simulink model "ModDem_OFDM_multicamino"  (R2018a)
settings: Solver=FixedStepAuto  StartTime=0.0  StopTime=M*CantBit  FixedStep=Tsampling  RelTol=1e-3
values from neighbouring files (symbols this model uses):
  EsOFDM = 2    [Script_configParametros_multicamino.m]
  F1 = FsepOFDM*2    [Script_configParametros_multicamino.m]
  F2 = FsepOFDM*3    [Script_configParametros_multicamino.m]
  F3 = FsepOFDM*4    [Script_configParametros_multicamino.m]
  F4 = FsepOFDM*5    [Script_configParametros_multicamino.m]
  RbOFDM = RsOFDM*sum(TransfBitPerSimb)    [Script_configParametros_multicamino.m]
  Ts1 = Tb1    (= 0.04)    [Script_configParametros_multicamino.m]
  Ts2 = Tb2    (= 0.04)    [Script_configParametros_multicamino.m]
  Ts3 = Tb3    (= 0.04)    [Script_configParametros_multicamino.m]
  Ts4 = Tb4    (= 0.04)    [Script_configParametros_multicamino.m]
  Tsampling = M/N    [Script_configParametros_multicamino.m]
libraries: commdigbbndpm3 x8, dspsigops x8, simulink x1, commrandsrc3 x1
settings Model: Creator=lukit  LastModifiedBy=geroo
settings DebuggingCC: LibraryContextMissingDiagnostic=warning
settings SFSimCC: SimUseLocalCustomCode=on
settings RTWCC: RTWUseLocalCustomCode=on

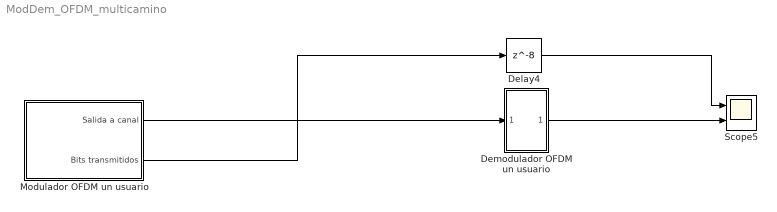
== system ModDem_OFDM_multicamino ==
  Delay4 : Delay  DelayLength=8  InitialCondition=0  InputProcessing=Columns as channels (frame based)
  Demodulador OFDM un usuario : Subsystem
  Modulador OFDM un usuario : Subsystem
  Scope5 : Scope  NumInputPorts=2
  wires:
  Modulador OFDM un usuario/2(Bits transmitidos) -> Delay4/1
  Delay4/1 -> Scope5/1
  Modulador OFDM un usuario/1(Salida a canal) -> Demodulador OFDM un usuario/1(In1)
  Demodulador OFDM un usuario/1(Out1) -> Scope5/2

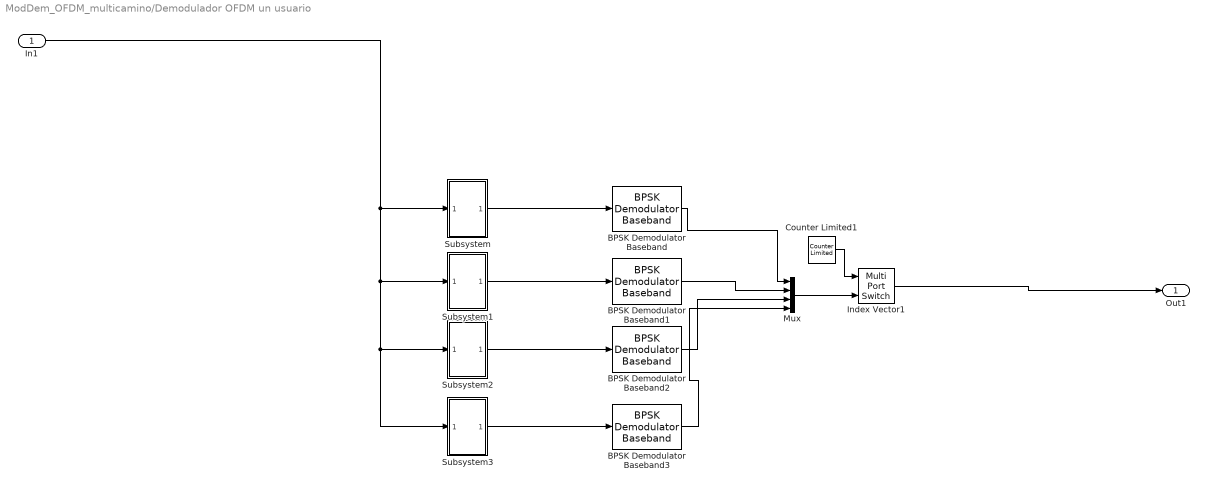
== system ModDem_OFDM_multicamino/Demodulador OFDM un usuario ==
  In1 : Inport
  BPSK Demodulator Baseband{,1..3} (4 alike) : commdigbbndpm3/BPSK Demodulator Baseband  DecType=Hard decision  VarSource=Dialog  Variance=1  Ph=0  outDtype=Inherit via internal rule  derotateFactorWordLen=16  derotateFactorDataTypeStr=Inherit: Same word length as input  derotateFactorLastDataTypeStr=Inherit: Same word length as input
  Counter Limited1 : simulink/Sources/Counter Limited  uplimit=3  tsamp=1/RbOFDM
  Index Vector1 : MultiPortSwitch  DataPortOrder=Zero-based contiguous  Inputs=1  zeroidx=on
  Mux : Mux
  Subsystem : Subsystem
  Subsystem1 : Subsystem
  Subsystem2 : Subsystem
  Subsystem3 : Subsystem
  Out1 : Outport
  wires:
  Subsystem1/1(Out1) -> BPSK Demodulator Baseband1/1
  Subsystem/1(Out1) -> BPSK Demodulator Baseband/1
  Index Vector1/1 -> Out1/1
  BPSK Demodulator Baseband3/1 -> Mux/4
  Subsystem2/1(Out1) -> BPSK Demodulator Baseband2/1
  In1/1 -> Subsystem3/1(In1), Subsystem2/1(In1), Subsystem1/1(In1), Subsystem/1(In1)
  BPSK Demodulator Baseband2/1 -> Mux/3
  BPSK Demodulator Baseband1/1 -> Mux/2
  BPSK Demodulator Baseband/1 -> Mux/1
  Mux/1 -> Index Vector1/2
  Subsystem3/1(Out1) -> BPSK Demodulator Baseband3/1
  Counter Limited1/1 -> Index Vector1/1

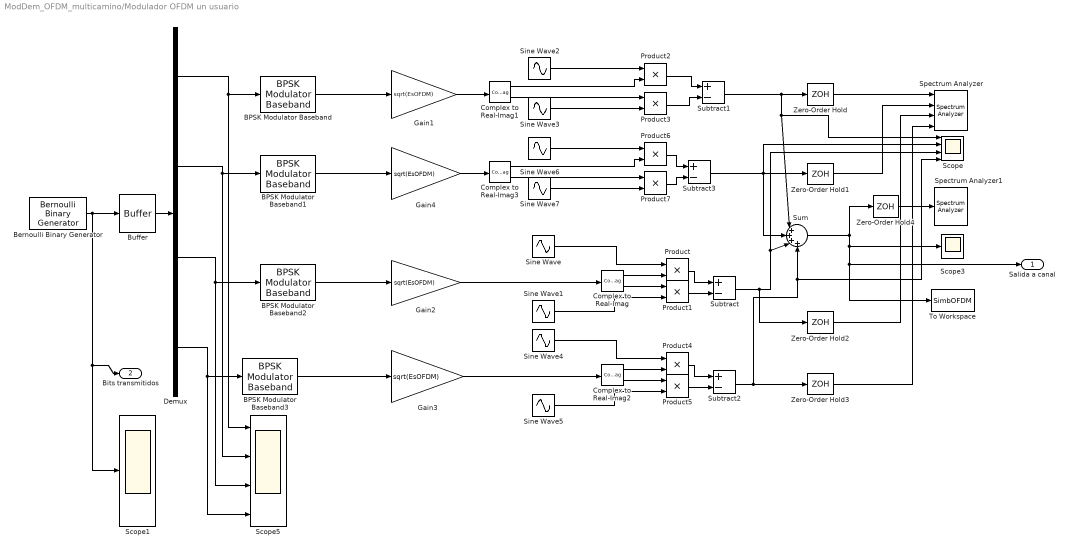
== system ModDem_OFDM_multicamino/Modulador OFDM un usuario ==
  BPSK Modulator Baseband{,1..3} (4 alike) : commdigbbndpm3/BPSK Modulator Baseband  Ph=0  outDtype=double  outWordLen=16  outUDDataType=sfix(16)  outFracLenMode=Best precision  outFracLen=15  outDataTypeStr=double  outLastDataTypeStr=double
  Bernoulli Binary Generator : commrandsrc3/Bernoulli Binary Generator  ProbabilityOfZero=0.5  SeedSource=Auto  Seed=0  SampleTime=1/RbOFDM  SamplesPerFrame=1  OutputDataType=double  SimulateUsing=Interpreted execution
  Buffer : Buffer  N=4  OutputFrames=off
  Complex to Real-Imag{,1..3} (4 alike) : ComplexToRealImag
  Demux : Demux
  Gain{1..4} (4 alike) : Gain  Gain=sqrt(EsOFDM)
  Product{,1..7} (8 alike) : Product
  Scope : Scope  NumInputPorts=4
  Scope1 : Scope
  Scope3 : Scope
  Scope5 : Scope  NumInputPorts=4
  Sine Wave : Sin  Amplitude=sqrt(2/Ts3)  Frequency=2*pi*F3  Phase=pi/2  SampleTime=Tsampling
  Sine Wave1 : Sin  Amplitude=sqrt(2/Ts3)  Frequency=2*pi*F3  SampleTime=Tsampling
  Sine Wave2 : Sin  Amplitude=sqrt(2/Ts1)  Frequency=2*pi*F1  Phase=pi/2  SampleTime=Tsampling
  Sine Wave3 : Sin  Amplitude=sqrt(2/Ts1)  Frequency=2*pi*F1  SampleTime=Tsampling
  Sine Wave4 : Sin  Amplitude=sqrt(2/Ts4)  Frequency=2*pi*F4  Phase=pi/2  SampleTime=Tsampling
  Sine Wave5 : Sin  Amplitude=sqrt(2/Ts4)  Frequency=2*pi*F4  SampleTime=Tsampling
  Sine Wave6 : Sin  Amplitude=sqrt(2/Ts2)  Frequency=2*pi*F2  Phase=pi/2  SampleTime=Tsampling
  Sine Wave7 : Sin  Amplitude=sqrt(2/Ts2)  Frequency=2*pi*F2  SampleTime=Tsampling
  Spectrum Analyzer : SpectrumAnalyzer  NumInputPorts=4
  Spectrum Analyzer1 : SpectrumAnalyzer
  Subtract{,1..3} (4 alike) : Sum  Inputs=+-
  Sum : Sum  Inputs=|++++
  To Workspace : ToWorkspace  VariableName=SimbOFDM  SampleTime=Tsampling
      settings: Save2DSignal=2-D array (concatenate along first dimension)
  Zero-Order Hold{,1..4} (5 alike) : ZeroOrderHold  SampleTime=-1
  Salida a canal : Outport
  Bits transmitidos : Outport  Port=2
  wires:
  BPSK Modulator Baseband/1 -> Gain1/1
  Zero-Order Hold1/1 -> Spectrum Analyzer/2
  Complex to Real-Imag3/2 -> Product7/1
  Gain4/1 -> Complex to Real-Imag3/1
  Sine Wave5/1 -> Product5/2
  Gain1/1 -> Complex to Real-Imag1/1
  Bernoulli Binary Generator/1 -> Bits transmitidos/1, Scope1/1, Buffer/1
  Product/1 -> Subtract/1
  Complex to Real-Imag2/2 -> Product5/1
  Subtract3/1 -> Zero-Order Hold1/1, Sum/2, Scope/2
  Product2/1 -> Subtract1/1
  Subtract2/1 -> Zero-Order Hold3/1, Scope/4, Sum/4
  Zero-Order Hold2/1 -> Spectrum Analyzer/3
  Complex to Real-Imag1/2 -> Product3/1
  Sine Wave3/1 -> Product3/2
  Zero-Order Hold3/1 -> Spectrum Analyzer/4
  Gain2/1 -> Complex to Real-Imag/1
  Sine Wave2/1 -> Product2/1
  Demux/3 -> BPSK Modulator Baseband2/1, Scope5/3
  Subtract1/1 -> Sum/1, Scope/1, Zero-Order Hold/1
  Subtract/1 -> Zero-Order Hold2/1, Scope/3, Sum/3
  Product4/1 -> Subtract2/1
  Product3/1 -> Subtract1/2
  Buffer/1 -> Demux/1
  Sum/1 -> Salida a canal/1, To Workspace/1, Scope3/1, Zero-Order Hold4/1
  Product1/1 -> Subtract/2
  Sine Wave4/1 -> Product4/1
  Demux/1 -> BPSK Modulator Baseband/1, Scope5/1
  Complex to Real-Imag2/1 -> Product4/2
  Complex to Real-Imag/1 -> Product/2
  Sine Wave1/1 -> Product1/2
  Product7/1 -> Subtract3/2
  Zero-Order Hold4/1 -> Spectrum Analyzer1/1
  Demux/4 -> BPSK Modulator Baseband3/1, Scope5/4
  Sine Wave7/1 -> Product7/2
  Complex to Real-Imag1/1 -> Product2/2
  Zero-Order Hold/1 -> Spectrum Analyzer/1
  Complex to Real-Imag/2 -> Product1/1
  Sine Wave6/1 -> Product6/1
  Product6/1 -> Subtract3/1
  Sine Wave/1 -> Product/1
  BPSK Modulator Baseband3/1 -> Gain3/1
  BPSK Modulator Baseband2/1 -> Gain2/1
  Gain3/1 -> Complex to Real-Imag2/1
  Complex to Real-Imag3/1 -> Product6/2
  BPSK Modulator Baseband1/1 -> Gain4/1
  Product5/1 -> Subtract2/2
  Demux/2 -> BPSK Modulator Baseband1/1, Scope5/2

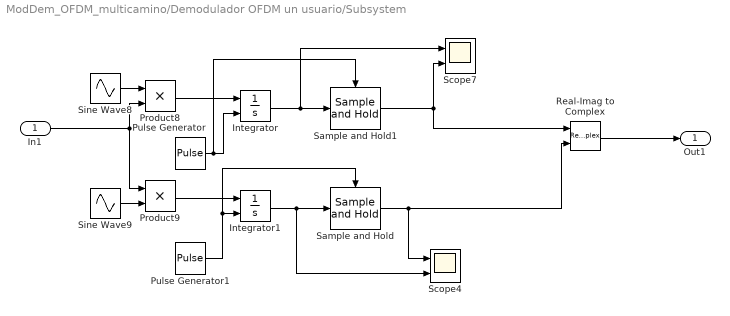
== system ModDem_OFDM_multicamino/Demodulador OFDM un usuario/Subsystem ==
  In1 : Inport
  Integrator : Integrator  ExternalReset=rising
  Integrator1 : Integrator  ExternalReset=rising
  Product8 : Product
  Product9 : Product
  Pulse Generator : DiscretePulseGenerator  PulseType=Time based  Period=Ts1  PulseWidth=99.9
  Pulse Generator1 : DiscretePulseGenerator  PulseType=Time based  Period=Ts1  PulseWidth=99.9
  Real-Imag to Complex : RealImagToComplex
  Sample and Hold : dspsigops/Sample and Hold  trig=Falling edge  initCond=0  latchinput=off
  Sample and Hold1 : dspsigops/Sample and Hold  trig=Falling edge  initCond=0  latchinput=off
  Scope4 : Scope  NumInputPorts=2
  Scope7 : Scope  NumInputPorts=2
  Sine Wave8 : Sin  Amplitude=sqrt(2/Ts1)  Frequency=2*pi*F1  Phase=pi/2  SampleTime=Tsampling
  Sine Wave9 : Sin  Amplitude=sqrt(2/Ts1)  Frequency=2*pi*F1  SampleTime=Tsampling
  Out1 : Outport
  wires:
  Product8/1 -> Integrator/1
  Integrator1/1 -> Scope4/2, Sample and Hold/1
  Product9/1 -> Integrator1/1
  Real-Imag to Complex/1 -> Out1/1
  Sine Wave8/1 -> Product8/1
  Sample and Hold/1 -> Real-Imag to Complex/2, Scope4/1
  Pulse Generator/1 -> Integrator/2, Sample and Hold1/Trigger
  Sample and Hold1/1 -> Scope7/2, Real-Imag to Complex/1
  Pulse Generator1/1 -> Integrator1/2, Sample and Hold/Trigger
  Sine Wave9/1 -> Product9/2
  Integrator/1 -> Scope7/1, Sample and Hold1/1
  In1/1 -> Product9/1, Product8/2

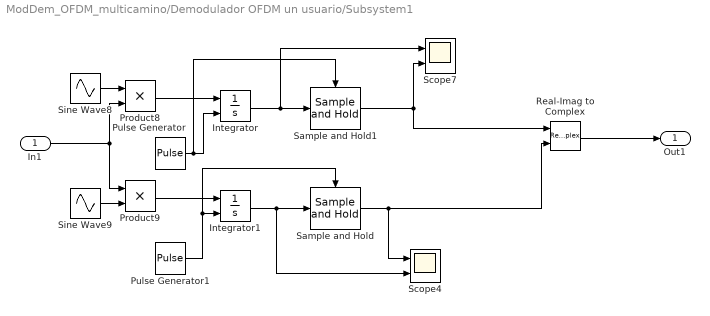
== system ModDem_OFDM_multicamino/Demodulador OFDM un usuario/Subsystem1 ==
  In1 : Inport
  Integrator : Integrator  ExternalReset=rising
  Integrator1 : Integrator  ExternalReset=rising
  Product8 : Product
  Product9 : Product
  Pulse Generator : DiscretePulseGenerator  PulseType=Time based  Period=Ts2  PulseWidth=99.9
  Pulse Generator1 : DiscretePulseGenerator  PulseType=Time based  Period=Ts2  PulseWidth=99.9
  Real-Imag to Complex : RealImagToComplex
  Sample and Hold : dspsigops/Sample and Hold  trig=Falling edge  initCond=0  latchinput=off
  Sample and Hold1 : dspsigops/Sample and Hold  trig=Falling edge  initCond=0  latchinput=off
  Scope4 : Scope  NumInputPorts=2
  Scope7 : Scope  NumInputPorts=2
  Sine Wave8 : Sin  Amplitude=sqrt(2/Ts2)  Frequency=2*pi*F2  Phase=pi/2  SampleTime=Tsampling
  Sine Wave9 : Sin  Amplitude=sqrt(2/Ts1)  Frequency=2*pi*F1  SampleTime=Tsampling
  Out1 : Outport
  wires:
  Product8/1 -> Integrator/1
  Integrator1/1 -> Scope4/2, Sample and Hold/1
  Product9/1 -> Integrator1/1
  Real-Imag to Complex/1 -> Out1/1
  Sine Wave8/1 -> Product8/1
  Sample and Hold/1 -> Real-Imag to Complex/2, Scope4/1
  Pulse Generator/1 -> Integrator/2, Sample and Hold1/Trigger
  Sample and Hold1/1 -> Scope7/2, Real-Imag to Complex/1
  Pulse Generator1/1 -> Integrator1/2, Sample and Hold/Trigger
  Sine Wave9/1 -> Product9/2
  Integrator/1 -> Scope7/1, Sample and Hold1/1
  In1/1 -> Product8/2, Product9/1

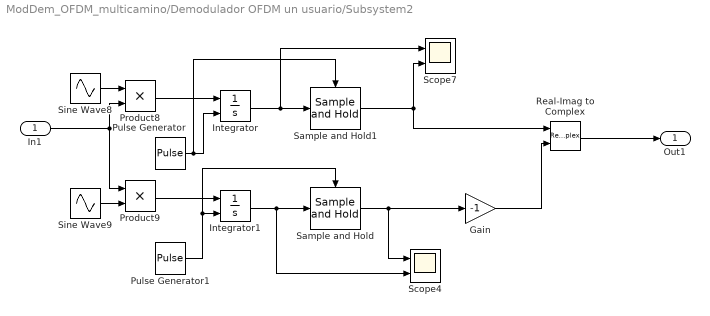
== system ModDem_OFDM_multicamino/Demodulador OFDM un usuario/Subsystem2 ==
  In1 : Inport
  Gain : Gain  Gain=-1
  Integrator : Integrator  ExternalReset=rising
  Integrator1 : Integrator  ExternalReset=rising
  Product8 : Product
  Product9 : Product
  Pulse Generator : DiscretePulseGenerator  PulseType=Time based  Period=Ts3  PulseWidth=99.9
  Pulse Generator1 : DiscretePulseGenerator  PulseType=Time based  Period=Ts3  PulseWidth=99.9
  Real-Imag to Complex : RealImagToComplex
  Sample and Hold : dspsigops/Sample and Hold  trig=Falling edge  initCond=0  latchinput=off
  Sample and Hold1 : dspsigops/Sample and Hold  trig=Falling edge  initCond=0  latchinput=off
  Scope4 : Scope  NumInputPorts=2
  Scope7 : Scope  NumInputPorts=2
  Sine Wave8 : Sin  Amplitude=sqrt(2/Ts3)  Frequency=2*pi*F3  Phase=pi/2  SampleTime=Tsampling
  Sine Wave9 : Sin  Amplitude=sqrt(2/Ts3)  Frequency=2*pi*F3  SampleTime=Tsampling
  Out1 : Outport
  wires:
  Product8/1 -> Integrator/1
  Integrator1/1 -> Scope4/2, Sample and Hold/1
  Product9/1 -> Integrator1/1
  Real-Imag to Complex/1 -> Out1/1
  Sine Wave8/1 -> Product8/1
  Sample and Hold/1 -> Gain/1, Scope4/1
  Pulse Generator/1 -> Integrator/2, Sample and Hold1/Trigger
  Sample and Hold1/1 -> Scope7/2, Real-Imag to Complex/1
  Pulse Generator1/1 -> Integrator1/2, Sample and Hold/Trigger
  Sine Wave9/1 -> Product9/2
  Integrator/1 -> Scope7/1, Sample and Hold1/1
  In1/1 -> Product9/1, Product8/2
  Gain/1 -> Real-Imag to Complex/2

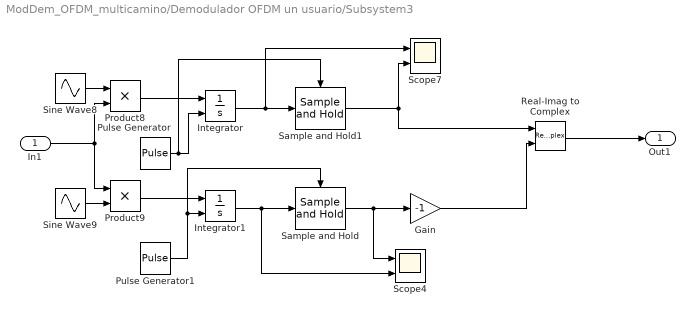
== system ModDem_OFDM_multicamino/Demodulador OFDM un usuario/Subsystem3 ==
  In1 : Inport
  Gain : Gain  Gain=-1
  Integrator : Integrator  ExternalReset=rising
  Integrator1 : Integrator  ExternalReset=rising
  Product8 : Product
  Product9 : Product
  Pulse Generator : DiscretePulseGenerator  PulseType=Time based  Period=Ts4  PulseWidth=99.9
  Pulse Generator1 : DiscretePulseGenerator  PulseType=Time based  Period=Ts4  PulseWidth=99.9
  Real-Imag to Complex : RealImagToComplex
  Sample and Hold : dspsigops/Sample and Hold  trig=Falling edge  initCond=0  latchinput=off
  Sample and Hold1 : dspsigops/Sample and Hold  trig=Falling edge  initCond=0  latchinput=off
  Scope4 : Scope  NumInputPorts=2
  Scope7 : Scope  NumInputPorts=2
  Sine Wave8 : Sin  Amplitude=sqrt(2/Ts4)  Frequency=2*pi*F4  Phase=pi/2  SampleTime=Tsampling
  Sine Wave9 : Sin  Amplitude=sqrt(2/Ts4)  Frequency=2*pi*F4  SampleTime=Tsampling
  Out1 : Outport
  wires:
  Product8/1 -> Integrator/1
  Integrator1/1 -> Scope4/2, Sample and Hold/1
  Product9/1 -> Integrator1/1
  Real-Imag to Complex/1 -> Out1/1
  Sine Wave8/1 -> Product8/1
  Sample and Hold/1 -> Gain/1, Scope4/1
  Pulse Generator/1 -> Integrator/2, Sample and Hold1/Trigger
  Sample and Hold1/1 -> Scope7/2, Real-Imag to Complex/1
  Pulse Generator1/1 -> Integrator1/2, Sample and Hold/Trigger
  Sine Wave9/1 -> Product9/2
  Integrator/1 -> Scope7/1, Sample and Hold1/1
  In1/1 -> Product8/2, Product9/1
  Gain/1 -> Real-Imag to Complex/2
